simulink model "Pressure_Controller_Test"  (R2026a)
settings: Solver=ode4  StopTime=60  FixedStep=P.sim.baseStep_s
undefined symbols (not defined in the file): CTRL, P
libraries: slpidlib x1
settings Model: Creator=jonat  LastModifiedBy=jonat

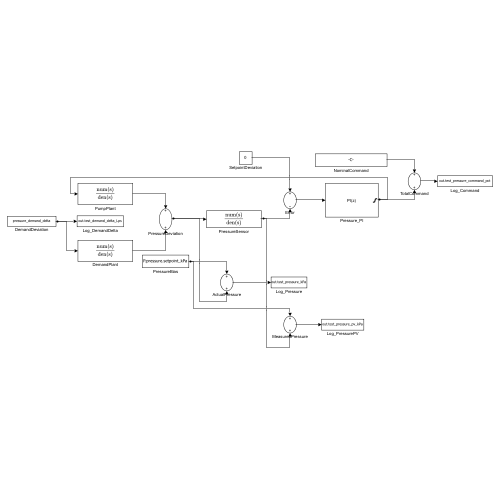
[thumbnail: Simulink's stored preview of the top-level diagram]
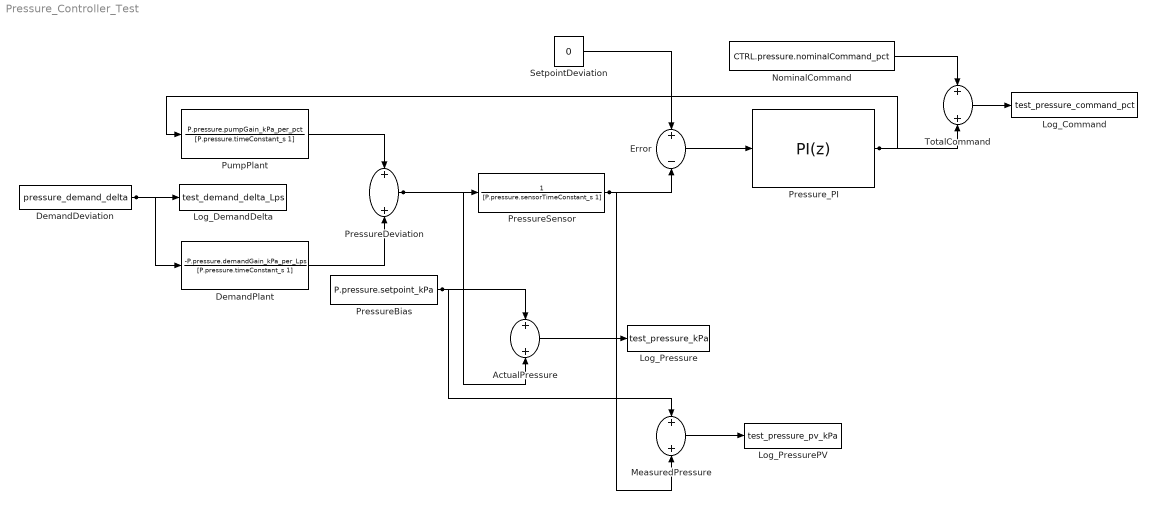
== system Pressure_Controller_Test ==
  ActualPressure : Sum
  DemandDeviation : FromWorkspace  VariableName=pressure_demand_delta  Interpolate=off  OutputAfterFinalValue=Holding final value
  DemandPlant : TransferFcn  Numerator=-P.pressure.demandGain_kPa_per_Lps  Denominator=[P.pressure.timeConstant_s 1]
  Error : Sum  Inputs=+-
  Log_Command : ToWorkspace  VariableName=test_pressure_command_pct  SaveFormat=Timeseries  SampleTime=-1
  Log_DemandDelta : ToWorkspace  VariableName=test_demand_delta_Lps  SaveFormat=Timeseries  SampleTime=-1
  Log_Pressure : ToWorkspace  VariableName=test_pressure_kPa  SaveFormat=Timeseries  SampleTime=-1
  Log_PressurePV : ToWorkspace  VariableName=test_pressure_pv_kPa  SaveFormat=Timeseries  SampleTime=-1
  MeasuredPressure : Sum
  NominalCommand : Constant  Value=CTRL.pressure.nominalCommand_pct
  PressureBias : Constant  Value=P.pressure.setpoint_kPa
  PressureDeviation : Sum
  PressureSensor : TransferFcn  Numerator=1  Denominator=[P.pressure.sensorTimeConstant_s 1]
  Pressure_PI : slpidlib/PID Controller  Controller=PI  Form=Parallel  TimeDomain=Discrete-time  UseExternalTs=off  SampleTime=CTRL.pressure.sampleTime_s  IntegratorMethod=Forward Euler  FilterMethod=Forward Euler  ControllerParametersSource=internal  P=CTRL.pressure.Kp  I=CTRL.pressure.Ki  UseKiTs=off  D=0  UseExternalDerivativeSource=off  N=100  UseFilter=on  TunerSelectOption=Transfer Function Based (PID Tuner App)  InitialConditionSource=internal  InitialConditionForIntegrator=0  InitialConditionForFilter=0  DifferentiatorICPrevScaledInput=0  ExternalReset=none  TrackingMode=off  Kt=1  LimitOutput=on  SatLimitsSource=internal  UpperSaturationLimit=CTRL.pressure.deltaOutputMax_pct  LowerSaturationLimit=CTRL.pressure.deltaOutputMin_pct  LinearizeAsGain=off  AntiWindupMode=clamping  Kb=1  LimitIntegrator=off  UpperIntegratorSaturationLimit=inf  LowerIntegratorSaturationLimit=-inf  POutMin=[]  POutMax=[]  IOutMin=[]  IOutMax=[]  DOutMin=[]  DOutMax=[]  NOutMin=[]  NOutMax=[]  SumOutMin=[]  SumOutMax=[]  SaturationOutMin=[]  SaturationOutMax=[]  PParamMin=[]  PParamMax=[]  IParamMin=[]  IParamMax=[]  DParamMin=[]  DParamMax=[]  NParamMin=[]  NParamMax=[]  KbParamMin=[]  KbParamMax=[]  KtParamMin=[]  KtParamMax=[]  KbOutMin=[]  KbOutMax=[]  KtOutMin=[]  KtOutMax=[]  IntegratorOutMin=[]  IntegratorOutMax=[]  FilterOutMin=[]  FilterOutMax=[]  SumI1OutMin=[]  SumI1OutMax=[]  SumI2OutMin=[]  SumI2OutMax=[]  SumI3OutMin=[]  SumI3OutMax=[]  SumI4OutMin=[]  SumI4OutMax=[]  SumDOutMin=[]  SumDOutMax=[]  DifferentiatorOutMin=[]  DifferentiatorOutMax=[]  FilterDiffOutCoefMin=[]  FilterDiffOutCoefMax=[]  ReciprocalOutMin=[]  ReciprocalOutMax=[]  SumDenOutMin=[]  SumDenOutMax=[]  SumNumOutMin=[]  SumNumOutMax=[]  DivideOutMin=[]  DivideOutMax=[]  UdiffTsProdOutMin=[]  UdiffTsProdOutMax=[]  NTsProdOutMin=[]  NTsProdOutMax=[]  UintegralTsProdOutMin=[]  UintegralTsProdOutMax=[]  UngainTsProdOutMin=[]  UngainTsProdOutMax=[]  ClampingZeroOutDataTypeStr=Inherit: Inherit via back propagation  ClampingZeroOutMin=[]  ClampingZeroOutMax=[]  FilterDenConstantOutDataTypeStr=Inherit: Inherit via back propagation  FilterDenConstantOutMin=[]  FilterDenConstantOutMax=[]  PCopyOutDataTypeStr=Inherit: Inherit via back propagation  PCopyOutMin=[]  PCopyOutMax=[]  NCopyOutDataTypeStr=Inherit: Inherit via back propagation  NCopyOutMin=[]  NCopyOutMax=[]  IntegratorContinuousStateAttributes=''  IntegratorStateMustResolveToSignalObject=off  IntegratorRTWStateStorageClass=Auto  FilterContinuousStateAttributes=''  FilterStateMustResolveToSignalObject=off  FilterRTWStateStorageClass=Auto  ParallelPVariant=InternalParameters  IdealPVariant=Disabled  IVariant=InternalParameters  DVariant=Disabled  IntegratorVariant=Discrete  SatVariant=Enabled  AWVariant=DiscClampingParallel  PCopyVariant=Disabled  TRVariant=Disabled  FdbkBlocksVariant=Forward  IdealPFdbkVariant=Disabled  SatFdbkVariant=Disabled  DerivativeFilterVariant=Disabled  NVariant=Disabled  NCopyVariant=Disabled_SignalSpec  FilterICVariant=Disabled  IntegratorICVariant=InternalICs  ExternalResetVariant=Disabled  TRSumVariant=Passthrough  SumFdbkVariant=Disabled  SumVariant=Sum_PI  TsampFilterVariant=InternalTs  TsampNgainVariant=Passthrough  TsampIntegralVariant=Disabled_SignalSpec  ExternalSaturationOutDataTypeStr=Inherit: Same as second input  DerivativeSourceVariant=Disabled  PreIntVariant=InternalPreInt
      settings: LibrarySourceBlock=simulink/Discrete/Discrete PID Controller
  PumpPlant : TransferFcn  Numerator=P.pressure.pumpGain_kPa_per_pct  Denominator=[P.pressure.timeConstant_s 1]
  SetpointDeviation : Constant  Value=0
  TotalCommand : Sum
  wires:
  DemandDeviation/1 -> DemandPlant/1, Log_DemandDelta/1
  ActualPressure/1 -> Log_Pressure/1
  PumpPlant/1 -> PressureDeviation/1
  DemandPlant/1 -> PressureDeviation/2
  PressureDeviation/1 -> ActualPressure/2, PressureSensor/1
  PressureBias/1 -> ActualPressure/1, MeasuredPressure/1
  PressureSensor/1 -> MeasuredPressure/2, Error/2
  NominalCommand/1 -> TotalCommand/1
  SetpointDeviation/1 -> Error/1
  Error/1 -> Pressure_PI/1
  MeasuredPressure/1 -> Log_PressurePV/1
  TotalCommand/1 -> Log_Command/1
  Pressure_PI/1 -> PumpPlant/1, TotalCommand/2
